simulink model "Satellite_simulink_linmod"  (R2018b)
settings: Solver=VariableStepAuto  StartTime=0.0  StopTime=10.0  RelTol=1e-3
values from neighbouring files (symbols this model uses):
  a = 0.5736    [Lab1.m]    (also in Micro_Sat_Open_Loop.m)
  J_s = 31.38    [Lab1.m]    (also in Micro_Sat_Open_Loop.m)
  w = 2.6268    [Lab1.m]    (also in Micro_Sat_Open_Loop.m)
settings Model: Creator=EKOCULU  LastModifiedBy=EKOCULU

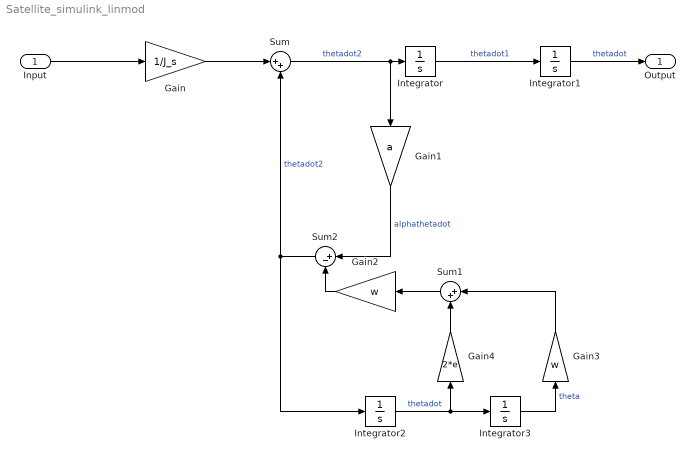
== system Satellite_simulink_linmod ==
  Input : Inport
  Gain : Gain  Gain=1/J_s
  Gain1 : Gain  Gain=a
  Gain2 : Gain  Gain=w
  Gain3 : Gain  Gain=w
  Gain4 : Gain  Gain=2*e
  Integrator{,1..3} (4 alike) : Integrator
  Sum : Sum  Inputs=|++
  Sum1 : Sum  Inputs=|++
  Sum2 : Sum  Inputs=|+-
  Output : Outport
  wires:
  Sum1/1 -> Gain2/1
  Sum/1 -> Gain1/1, Integrator/1  "thetadot2"
  Sum2/1 -> Integrator2/1, Sum/2  "thetadot2"
  Gain3/1 -> Sum1/1
  Integrator3/1 -> Gain3/1  "theta"
  Integrator1/1 -> Output/1  "thetadot"
  Gain/1 -> Sum/1
  Gain4/1 -> Sum1/2
  Integrator/1 -> Integrator1/1  "thetadot1"
  Integrator2/1 -> Gain4/1, Integrator3/1  "thetadot"
  Gain1/1 -> Sum2/1  "alphathetadot"
  Input/1 -> Gain/1
  Gain2/1 -> Sum2/2
